simulink model "ans15"  (R2019a)
settings: Solver=VariableStepAuto  StartTime=0.0  StopTime=10.0  RelTol=1e-3
undefined symbols (not defined in the file or in its folder): f_effi, J_effi, K_T, KD, KI, KP, n, qr_i, T_L
settings Model: Creator=andylei  LastModifiedBy=matth
settings DataIOCC: SaveFormat=StructureWithTime  ReturnWorkspaceOutputs=off
settings DebuggingCC: ArithmeticOperatorsInVariantConditions=warning

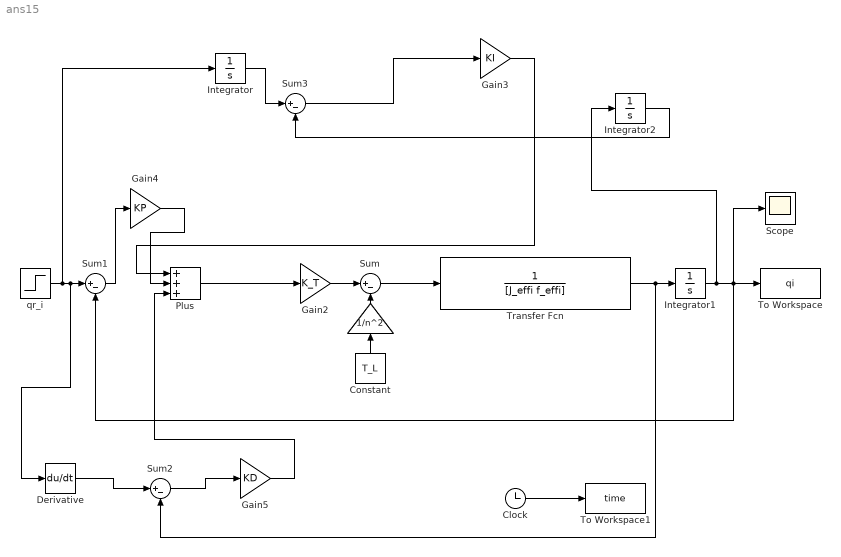
== system ans15 ==
  " " : Gain  Gain=1/n^2
  Clock : Clock
  Constant : Constant  Value=T_L
  Derivative : Derivative
  Gain2 : Gain  Gain=K_T
  Gain3 : Gain  Gain=KI
  Gain4 : Gain  Gain=KP
  Gain5 : Gain  Gain=KD
  Integrator : Integrator
  Integrator1 : Integrator
  Integrator2 : Integrator
  Plus : Sum  Inputs=+++
  Scope : Scope
  Sum{,1..3} (4 alike) : Sum  Inputs=|+-
  To Workspace : ToWorkspace  VariableName=qi  SampleTime=-1
  To Workspace1 : ToWorkspace  VariableName=time  SampleTime=-1
  Transfer Fcn : TransferFcn  Denominator=[J_effi f_effi]
  qr_i : Step  Before=qr_i  After=qr_i  SampleTime=0
  wires:
  Transfer Fcn/1 -> Sum2/2, Integrator1/1
  Sum/1 -> Transfer Fcn/1
  Constant/1 -> " "/1
  " "/1 -> Sum/2
  Gain2/1 -> Sum/1
  Clock/1 -> To Workspace1/1
  Plus/1 -> Gain2/1
  Sum1/1 -> Gain4/1
  Gain4/1 -> Plus/2
  Integrator1/1 -> Integrator2/1, To Workspace/1, Scope/1, Sum1/2
  qr_i/1 -> Integrator/1, Derivative/1, Sum1/1
  Derivative/1 -> Sum2/1
  Sum2/1 -> Gain5/1
  Gain5/1 -> Plus/3
  Integrator2/1 -> Sum3/2
  Integrator/1 -> Sum3/1
  Sum3/1 -> Gain3/1
  Gain3/1 -> Plus/1
